simulink model "a04_standartregelkreis_part_c"  (R2018a)
settings: Solver=VariableStepAuto  StartTime=0.0  StopTime=10.0  RelTol=1e-3
settings Model: Creator=oleksandra  LastModifiedBy=oleksandra

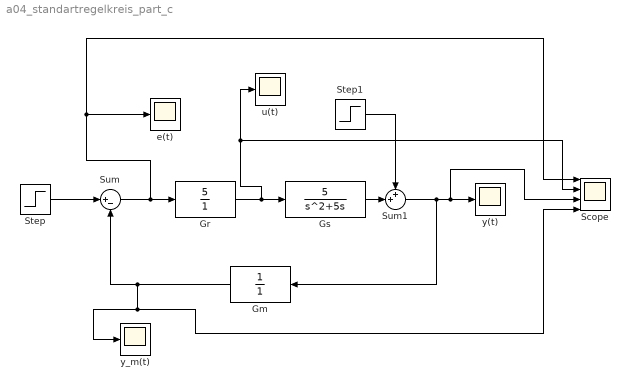
== system a04_standartregelkreis_part_c ==
  Gm : TransferFcn  Denominator=[1]
  Gr : TransferFcn  Numerator=[5]  Denominator=[1]
  Gs : TransferFcn  Numerator=[0 0 5]  Denominator=[1 5 0]
  Scope : Scope  NumInputPorts=4
  Step : Step  Time=0  After=5  SampleTime=0
  Step1 : Step  Time=2  After=6  SampleTime=0
  Sum : Sum  Inputs=|+-
  Sum1 : Sum  Inputs=++|
  e(t) : Scope
  u(t) : Scope
  y(t) : Scope
  y_m(t) : Scope
  wires:
  Step/1 -> Sum/1
  Sum/1 -> Scope/1, e(t)/1, Gr/1
  Gr/1 -> Scope/2, u(t)/1, Gs/1
  Gs/1 -> Sum1/2
  Step1/1 -> Sum1/1
  Gm/1 -> Scope/4, y_m(t)/1, Sum/2
  Sum1/1 -> Gm/1, Scope/3, y(t)/1
